simulink model "encoder_slsp_mega"  (Simulink 8.0)
settings: Solver=FixedStepDiscrete  SolverMode=SingleTasking  StartTime=0.0  StopTime=10.0  RelTol=1e-3
settings Model: Creator=gcampa  LastModifiedBy=gcampa  ExtModeTrigDuration=2
settings DataIOCC: SignalLoggingSaveFormat=ModelDataLogs  SaveOutput=off  SaveTime=off
settings OptimizationCC: OptimizeModelRefInitCode=on  LifeSpan=1
settings DebuggingCC: SolverPrmCheckMsg=none  FcnCallInpInsideContextMsg=EnableAllAsWarning  StrictBusMsg=Warning
settings HardwareCC: ProdBitPerInt=16  ProdBitPerPointer=16  ProdIntDivRoundTo=Zero  ProdEndianess=LittleEndian  ProdWordSize=8  ProdHWDeviceType=Atmel->AVR
settings RTWCC: SystemTargetFile=realtime.tlc  GenerateMakefile=off  TemplateMakefile=realtime.tmf  Description=Real-Time Toolbox  RTWVerbose=off  ProcessScript=realtime_make_rtw_hook
settings STFCustomTargetCC: TargetLibSuffix=.a  CodeReplacementLibrary=ANSI_C  GenerateSampleERTMain=on  ERTCustomFileBanners=on  SupportNonInlinedSFcns=off  SupportVariableSizeSignals=on  GRTInterface=off  SystemTargetFile=realtime.tlc
settings ERTTargetCC: CodeReplacementLibrary=ANSI_C  MultiwordLength=2048  GenerateSampleERTMain=on  ParMdlRefBuildCompliant=off  CompOptLevelCompliant=off  ConcurrentExecutionCompliant=off  CombineOutputUpdateFcns=off  ERTFirstTimeCompliant=off  SupportContinuousTime=on  SupportVariableSizeSignals=on  ModelStepFunctionPrototypeControlCompliant=off  CPPClassGenCompliant=off  ExtModeTransport=3  ExtModeMexFile=ext_serial_win32_comm  ExtModeMexArgs=0 1 9600  InlinedParameterPlacement=NonHierarchical  ERTSrcFileBannerTemplate=realtime_code_template.cgt  ERTHdrFileBannerTemplate=realtime_code_template.cgt  ERTDataSrcFileTemplate=realtime_code_template.cgt  ERTDataHdrFileTemplate=realtime_code_template.cgt  ERTCustomFileTemplate=realtime_file_process.tlc  ConvertIfToSwitch=off  SuppressUnreachableDefaultCases=off
settings SettingsController: Description=Run on Hardware Dialog  TargetExtensionPlatform=Arduino Mega 2560
settings MATStruct: Set_host_COM_port=[0.0]  COM_port_number=1  COM_port_baud_rate=115200  Enable_overrun_detection=[0.0]  Digital_output_to_set_on_overrun=13  Analog_input_reference_voltage=[0.0]  Serial0_baud_rate=9600  Serial1_baud_rate=9600  Serial2_baud_rate=9600  Serial3_baud_rate=9600

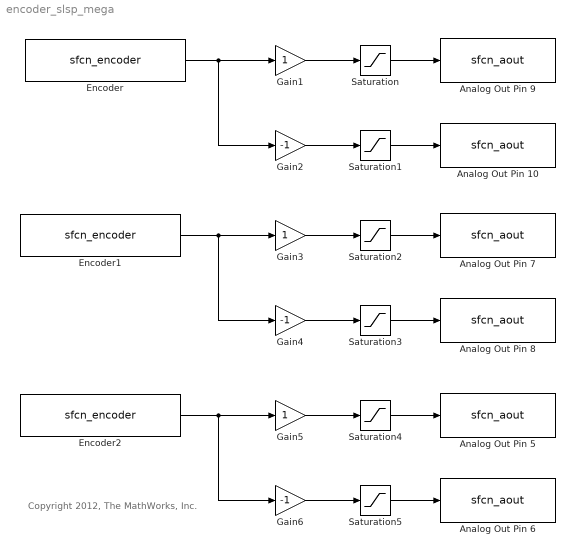
== system encoder_slsp_mega ==
  note: Copyright 2012, The MathWorks, Inc.
  Analog Out Pin 10 : S-Function  InitFcn=try, set_param(gcb,'FunctionName','sfcn_aout'), end  FunctionName=sfcn_aout  Parameters=uint8(10)  SFunctionModules=sfcn_aout_wrapper  WizardData=DataTag0  EnableBusSupport=off  mask(S-Function Builder){}
      mask init:
      | val = [[.9  0.75 0.75 1 1 .9 .9 1]',[1 1 0.75 0.75 .9 .9 1 .9]'];try , sys = get_param(gcb,'SfunBuilderFcnName');if isempty(sys), sys = get_param(gcb,'FunctionName'); end,catch, sys = get_param(gcb,'FunctionName'); end
      settings: CopyFcn=set_param(gcbh,'LinkStatus','none')  PreSaveFcn=try, set_param(gcb,'FunctionName','sfcn_aout'), end  OpenFcn=sfunctionwizard(gcbh)
      mask Display: plot(val(:,1),val(:,2)),disp(sys), port_label('input',1,'in')
  Analog Out Pin 5 : S-Function  InitFcn=try, set_param(gcb,'FunctionName','sfcn_aout'), end  FunctionName=sfcn_aout  Parameters=uint8(5)  SFunctionModules=sfcn_aout_wrapper  WizardData=DataTag1  EnableBusSupport=off  mask(S-Function Builder){}
      mask init: same as encoder_slsp_mega/Analog Out Pin 10
      settings: CopyFcn=set_param(gcbh,'LinkStatus','none')  PreSaveFcn=try, set_param(gcb,'FunctionName','sfcn_aout'), end  OpenFcn=sfunctionwizard(gcbh)
      mask Display: plot(val(:,1),val(:,2)),disp(sys), port_label('input',1,'in')
  Analog Out Pin 6 : S-Function  InitFcn=try, set_param(gcb,'FunctionName','sfcn_aout'), end  FunctionName=sfcn_aout  Parameters=uint8(6)  SFunctionModules=sfcn_aout_wrapper  WizardData=DataTag2  EnableBusSupport=off  mask(S-Function Builder){}
      mask init: same as encoder_slsp_mega/Analog Out Pin 10
      settings: CopyFcn=set_param(gcbh,'LinkStatus','none')  PreSaveFcn=try, set_param(gcb,'FunctionName','sfcn_aout'), end  OpenFcn=sfunctionwizard(gcbh)
      mask Display: plot(val(:,1),val(:,2)),disp(sys), port_label('input',1,'in')
  Analog Out Pin 7 : S-Function  InitFcn=try, set_param(gcb,'FunctionName','sfcn_aout'), end  FunctionName=sfcn_aout  Parameters=uint8(7)  SFunctionModules=sfcn_aout_wrapper  WizardData=DataTag3  EnableBusSupport=off  mask(S-Function Builder){}
      mask init: same as encoder_slsp_mega/Analog Out Pin 10
      settings: CopyFcn=set_param(gcbh,'LinkStatus','none')  PreSaveFcn=try, set_param(gcb,'FunctionName','sfcn_aout'), end  OpenFcn=sfunctionwizard(gcbh)
      mask Display: plot(val(:,1),val(:,2)),disp(sys), port_label('input',1,'in')
  Analog Out Pin 8 : S-Function  InitFcn=try, set_param(gcb,'FunctionName','sfcn_aout'), end  FunctionName=sfcn_aout  Parameters=uint8(8)  SFunctionModules=sfcn_aout_wrapper  WizardData=DataTag4  EnableBusSupport=off  mask(S-Function Builder){}
      mask init: same as encoder_slsp_mega/Analog Out Pin 10
      settings: CopyFcn=set_param(gcbh,'LinkStatus','none')  PreSaveFcn=try, set_param(gcb,'FunctionName','sfcn_aout'), end  OpenFcn=sfunctionwizard(gcbh)
      mask Display: plot(val(:,1),val(:,2)),disp(sys), port_label('input',1,'in')
  Analog Out Pin 9 : S-Function  InitFcn=try, set_param(gcb,'FunctionName','sfcn_aout'), end  FunctionName=sfcn_aout  Parameters=uint8(9)  SFunctionModules=sfcn_aout_wrapper  WizardData=DataTag5  EnableBusSupport=off  mask(S-Function Builder){}
      mask init: same as encoder_slsp_mega/Analog Out Pin 10
      settings: CopyFcn=set_param(gcbh,'LinkStatus','none')  PreSaveFcn=try, set_param(gcb,'FunctionName','sfcn_aout'), end  OpenFcn=sfunctionwizard(gcbh)
      mask Display: plot(val(:,1),val(:,2)),disp(sys), port_label('input',1,'in')
  Encoder : S-Function  InitFcn=try, set_param(gcb,'FunctionName','sfcn_encoder'), end  FunctionName=sfcn_encoder  Parameters=uint8(0),uint8(2),uint8(3)  SFunctionModules=sfcn_encoder_wrapper  WizardData=DataTag6  EnableBusSupport=off  mask(S-Function Builder){}
      mask init: same as encoder_slsp_mega/Analog Out Pin 10
      settings: CopyFcn=set_param(gcbh,'LinkStatus','none')  PreSaveFcn=try, set_param(gcb,'FunctionName','sfcn_encoder'), end  OpenFcn=sfunctionwizard(gcbh)
      mask Display: plot(val(:,1),val(:,2)),disp(sys), port_label('output',1,'pos')
  Encoder1 : S-Function  InitFcn=try, set_param(gcb,'FunctionName','sfcn_encoder'), end  FunctionName=sfcn_encoder  Parameters=uint8(1),uint8(18),uint8(19)  SFunctionModules=sfcn_encoder_wrapper  WizardData=DataTag7  EnableBusSupport=off  mask(S-Function Builder){}
      mask init: same as encoder_slsp_mega/Analog Out Pin 10
      settings: CopyFcn=set_param(gcbh,'LinkStatus','none')  PreSaveFcn=try, set_param(gcb,'FunctionName','sfcn_encoder'), end  OpenFcn=sfunctionwizard(gcbh)
      mask Display: plot(val(:,1),val(:,2)),disp(sys), port_label('output',1,'pos')
  Encoder2 : S-Function  InitFcn=try, set_param(gcb,'FunctionName','sfcn_encoder'), end  FunctionName=sfcn_encoder  Parameters=uint8(2),uint8(20),uint8(21)  SFunctionModules=sfcn_encoder_wrapper  WizardData=DataTag8  EnableBusSupport=off  mask(S-Function Builder){}
      mask init: same as encoder_slsp_mega/Analog Out Pin 10
      settings: CopyFcn=set_param(gcbh,'LinkStatus','none')  PreSaveFcn=try, set_param(gcb,'FunctionName','sfcn_encoder'), end  OpenFcn=sfunctionwizard(gcbh)
      mask Display: plot(val(:,1),val(:,2)),disp(sys), port_label('output',1,'pos')
  Gain1 : Gain  OutDataTypeStr=Inherit: Same as input
  Gain2 : Gain  Gain=-1  OutDataTypeStr=Inherit: Same as input
  Gain3 : Gain  OutDataTypeStr=Inherit: Same as input
  Gain4 : Gain  Gain=-1  OutDataTypeStr=Inherit: Same as input
  Gain5 : Gain  OutDataTypeStr=Inherit: Same as input
  Gain6 : Gain  Gain=-1  OutDataTypeStr=Inherit: Same as input
  Saturation{,1..5} (6 alike) : Saturate  UpperLimit=255  LowerLimit=0  OutDataTypeStr=uint8
  wires:
  Gain2/1 -> Saturation1/1
  Encoder/1 -> Gain2/1, Gain1/1
  Gain1/1 -> Saturation/1
  Saturation/1 -> Analog Out Pin 9/1
  Saturation1/1 -> Analog Out Pin 10/1
  Gain4/1 -> Saturation3/1
  Encoder1/1 -> Gain3/1, Gain4/1
  Gain3/1 -> Saturation2/1
  Saturation2/1 -> Analog Out Pin 7/1
  Saturation3/1 -> Analog Out Pin 8/1
  Gain6/1 -> Saturation5/1
  Encoder2/1 -> Gain6/1, Gain5/1
  Gain5/1 -> Saturation4/1
  Saturation4/1 -> Analog Out Pin 5/1
  Saturation5/1 -> Analog Out Pin 6/1
